simulink model "motor_identification_2021_MATLAB"  (R2021b)
settings: Solver=ode5  StartTime=0.0  StopTime=inf  FixedStep=0.01  RelTol=1e-3
libraries: instrumentseriallib x2, etargetslib x1
settings Model: Creator=arian  LastModifiedBy=arian
settings DebuggingCC: UnconnectedInputMsg=none  UnconnectedOutputMsg=none  UnconnectedLineMsg=none
settings HardwareCC: ProdBitPerLong=64  ProdHWDeviceType=Intel->x86-64 (Linux 64)
settings ModelReferenceCC: EnableRefExpFcnMdlSchedulingChecks=off
settings RTWCC: Description=Simulink Desktop Real-Time  SystemTargetFile=sldrt.tlc  TemplateMakefile=sldrt.tmf  RTWCompilerOptimization=on  DLArmComputeVersion=20.02.1
settings CodeAppCC: MaxIdLength=95
settings SimulinkDesktopRealTimeCC: TargetLibSuffix=_sldrt.a  TargetPreCompLibLocation=C:\Program Files\MATLAB\R2023a\toolbox\sldrt\lib\win64

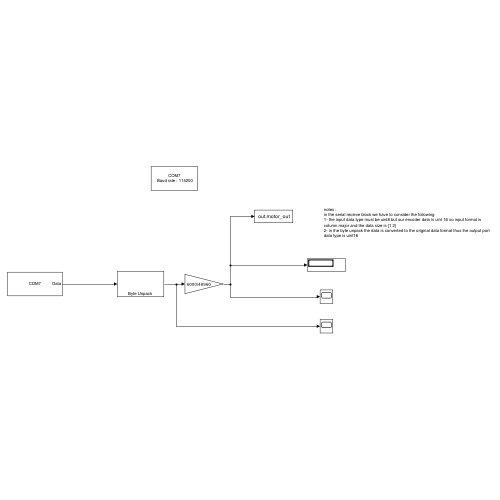
[thumbnail: Simulink's stored preview of the top-level diagram]
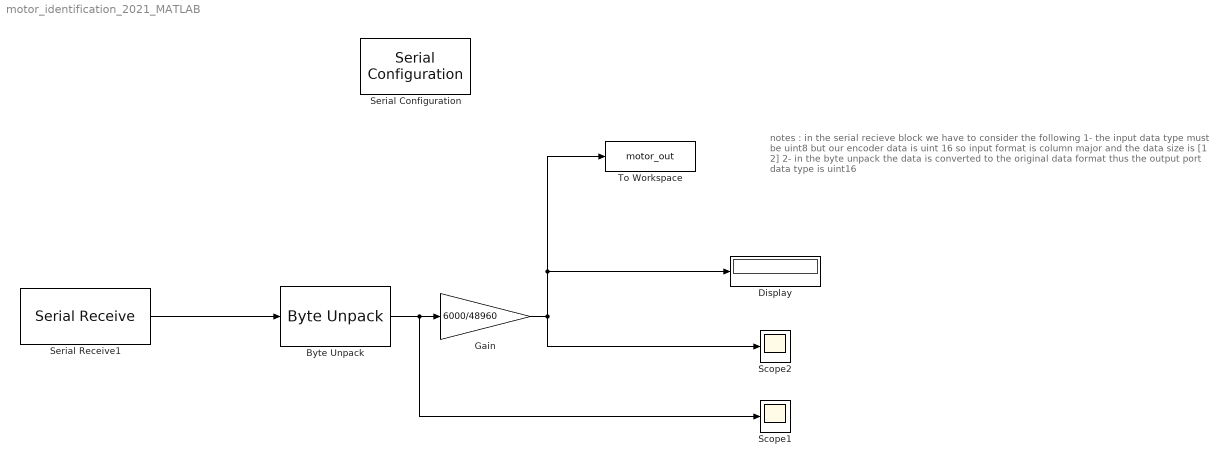
== system motor_identification_2021_MATLAB ==
  note: notes :
      | in the serial recieve block we have to consider the following
      | 1- the input data type must be uint8 but our encoder data is uint 16 so input format is column major and the data size is [1 2]
      | 2- in the byte unpack the data is converted to the original data format thus the output port data type is uint16
  Byte Unpack : etargetslib/Byte Unpack  dimensions={[1]}  datatypes={'uint16'}  byteAlign=1
  Display : Display
  Gain : Gain  Gain=6000/48960
  Scope1 : Scope
  Scope2 : Scope
  Serial Configuration : instrumentseriallib/Serial Configuration  Priority=-200000  Port=COM7  ComPort=COM7  BaudRate=115200  DataBits=8  Parity=none  StopBits=1  ByteOrder=little-endian  FlowControl=none  Timeout=10  SimulateUsing=Interpreted execution  BlockInModel=on
  Serial Receive1 : instrumentseriallib/Serial Receive  Priority=1  Port=COM7  ComPort=COM7  DataType=uint8  SaveDataType=uint8  ToggleHeader=off  Header=[]  ToggleTerminator=off  Terminator=<none>  CustomTerminator=[]  ToggleDataSize=on  DataSize=[1 2]  EnableBlockingMode=on  ActionDataUnavailable=Output last received value  ActionWhenDataUnavailable=Output last received value  CustomValue=0  SampleTime=0.01  SimulateUsing=Interpreted execution  BlockInModel=on
  To Workspace : ToWorkspace  VariableName=motor_out  SaveFormat=Timeseries  SampleTime=-1
  wires:
  Serial Receive1/1 -> Byte Unpack/1
  Gain/1 -> Scope2/1, To Workspace/1, Display/1
  Byte Unpack/1 -> Scope1/1, Gain/1
